simulink model "PC_MSFS_STATION"  (R2021b)
settings: Solver=FixedStepAuto  StartTime=0.0  StopTime=600  FixedStep=0.03  RelTol=1e-3
undefined symbols (not defined in the file): DiscIntNeverNeededParam, MODEL, MODEL_INI
libraries: SimConnectToolbox x9, simulink x4
(part 1 of 2)
settings Model: Creator=Andreas  LastModifiedBy=ccortes9
settings SolverCC: AlgebraicLoopSolver=TrustRegion
settings DebuggingCC: InheritedTsInSrcMsg=none  SFMachineParentedDataDiag=warning

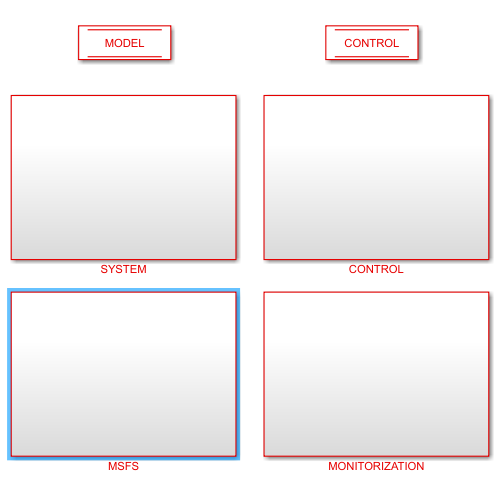
[thumbnail: Simulink's stored preview of the top-level diagram]
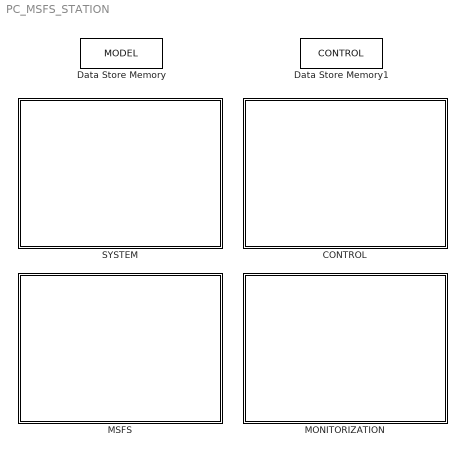
== system PC_MSFS_STATION ==
  CONTROL : Subsystem
  Data Store Memory : DataStoreMemory  DataStoreName=MODEL  ReadBeforeWriteMsg=warning  WriteAfterWriteMsg=warning  WriteAfterReadMsg=warning  InitialValue=MODEL_INI  ShowAdditionalParam=off  OutDataTypeStr=Bus: MODEL_Bus
  Data Store Memory1 : DataStoreMemory  DataStoreName=CONTROL  ReadBeforeWriteMsg=warning  WriteAfterWriteMsg=warning  WriteAfterReadMsg=warning  InitialValue=CONTROL_INI  ShowAdditionalParam=off  OutDataTypeStr=Bus: CONTROL_Bus
  MONITORIZATION : Subsystem
  MSFS : Subsystem
  SYSTEM : Subsystem

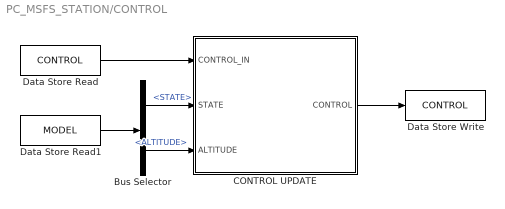
== system PC_MSFS_STATION/CONTROL ==
  Bus Selector : BusSelector  OutputSignals=STATE,INPUT.ALTITUDE
  CONTROL UPDATE : MATLAB Function  TreatAsAtomicUnit=on
  Data Store Read : DataStoreRead  DataStoreName=CONTROL  SampleTime=MODEL_INI.PARAM.SIM_SAMPLING_TIME  IndexOptions=Index vector (dialog)  Indices=1  OutputSizes=1
  Data Store Read1 : DataStoreRead  DataStoreName=MODEL  SampleTime=MODEL_INI.PARAM.SIM_SAMPLING_TIME  IndexOptions=Index vector (dialog)  Indices=1  OutputSizes=1
  Data Store Write : DataStoreWrite  DataStoreName=CONTROL  IndexOptions=Index vector (dialog)  Indices=1  OutputSizes=1
  wires:
  Data Store Read/1 -> CONTROL UPDATE/1(CONTROL_IN)
  CONTROL UPDATE/1(CONTROL) -> Data Store Write/1
  Bus Selector/1 -> CONTROL UPDATE/2(STATE)  "<STATE>"
  Data Store Read1/1 -> Bus Selector/1
  Bus Selector/2 -> CONTROL UPDATE/3(ALTITUDE)  "<ALTITUDE>"

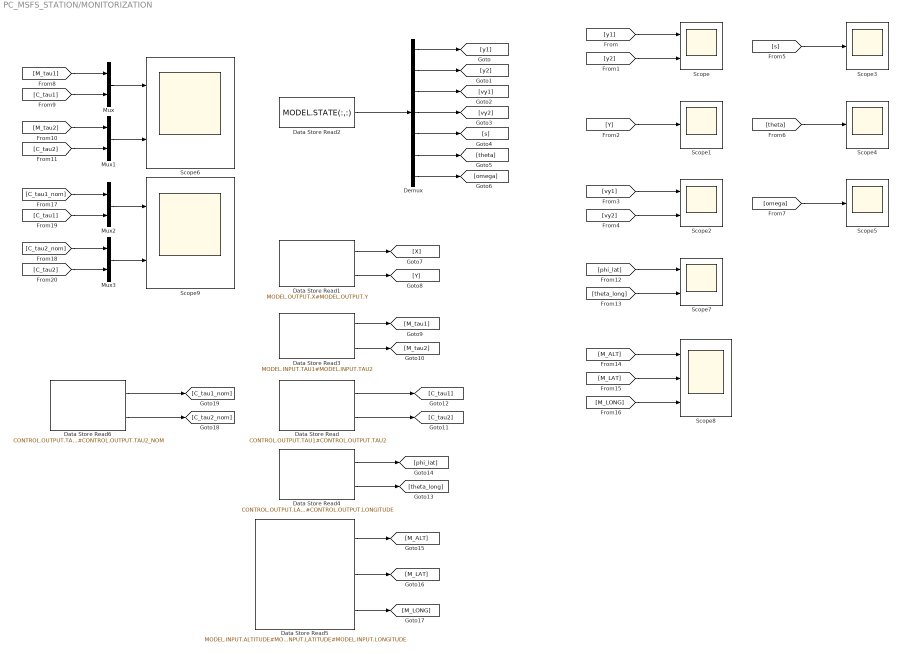
== system PC_MSFS_STATION/MONITORIZATION ==
  Data Store Read : DataStoreRead  DataStoreName=CONTROL  DataStoreElements=CONTROL.OUTPUT.TAU1#CONTROL.OUTPUT.TAU2  IndexOptions=Index vector (dialog)  Indices=1  OutputSizes=1
  Data Store Read1 : DataStoreRead  DataStoreName=MODEL  SampleTime=MODEL_INI.PARAM.SIM_SAMPLING_TIME  DataStoreElements=MODEL.OUTPUT.X#MODEL.OUTPUT.Y  IndexOptions=Index vector (dialog)  Indices=1  OutputSizes=1
  Data Store Read2 : DataStoreRead  DataStoreName=MODEL  SampleTime=MODEL_INI.PARAM.SIM_SAMPLING_TIME  DataStoreElements=MODEL.STATE(:,:)  IndexOptions=Index vector (dialog)  Indices=1  OutputSizes=1
  Data Store Read3 : DataStoreRead  DataStoreName=MODEL  SampleTime=MODEL_INI.PARAM.SIM_SAMPLING_TIME  DataStoreElements=MODEL.INPUT.TAU1#MODEL.INPUT.TAU2  IndexOptions=Index vector (dialog)  Indices=1  OutputSizes=1
  Data Store Read4 : DataStoreRead  DataStoreName=CONTROL  DataStoreElements=CONTROL.OUTPUT.LATITUDE#CONTROL.OUTPUT.LONGITUDE  IndexOptions=Index vector (dialog)  Indices=1  OutputSizes=1
  Data Store Read5 : DataStoreRead  DataStoreName=MODEL  SampleTime=MODEL_INI.PARAM.SIM_SAMPLING_TIME  DataStoreElements=MODEL.INPUT.ALTITUDE#MODEL.INPUT.LATITUDE#MODEL.INPUT.LONGITUDE  IndexOptions=Index vector (dialog)  Indices=1  OutputSizes=1
  Data Store Read6 : DataStoreRead  DataStoreName=CONTROL  DataStoreElements=CONTROL.OUTPUT.TAU1_NOM#CONTROL.OUTPUT.TAU2_NOM  IndexOptions=Index vector (dialog)  Indices=1  OutputSizes=1
  Demux : Demux  Outputs=7
  Mux{,1..3} (4 alike) : Mux  Inputs=2
  Scope{,2,6..7,9} (5 alike) : Scope  NumInputPorts=2
  Scope{1,3..5} (4 alike) : Scope
  Scope8 : Scope  NumInputPorts=3
  wires:
  Data Store Read2/1 -> Demux/1
  Demux/1 -> [y1]
  Demux/2 -> [y2]
  Demux/3 -> [vy1]
  Demux/4 -> [vy2]
  Demux/5 -> [s]
  Demux/6 -> [theta]
  Demux/7 -> [omega]
  [y1] -> Scope/1
  [y2] -> Scope/2
  Data Store Read1/1 -> [X]
  Data Store Read1/2 -> [Y]
  [Y] -> Scope1/1
  [vy2] -> Scope2/2
  [vy1] -> Scope2/1
  [s] -> Scope3/1
  [theta] -> Scope4/1
  [omega] -> Scope5/1
  Data Store Read3/1 -> [M_tau1]
  Data Store Read3/2 -> [M_tau2]
  Data Store Read/1 -> [C_tau1]
  Data Store Read/2 -> [C_tau2]
  Mux/1 -> Scope6/1
  Mux1/1 -> Scope6/2
  [M_tau1] -> Mux/1
  [M_tau2] -> Mux1/1
  [C_tau2] -> Mux1/2
  [C_tau1] -> Mux/2
  [phi_lat] -> Scope7/1
  [theta_long] -> Scope7/2
  Data Store Read4/2 -> [theta_long]
  Data Store Read4/1 -> [phi_lat]
  Data Store Read5/2 -> [M_LAT]
  Data Store Read5/1 -> [M_ALT]
  Data Store Read5/3 -> [M_LONG]
  [M_LAT] -> Scope8/2
  [M_ALT] -> Scope8/1
  [M_LONG] -> Scope8/3
  Data Store Read6/2 -> [C_tau2_nom]
  Data Store Read6/1 -> [C_tau1_nom]
  [C_tau1] -> Mux2/2
  [C_tau2] -> Mux3/2
  [C_tau2_nom] -> Mux3/1
  [C_tau1_nom] -> Mux2/1
  Mux3/1 -> Scope9/2
  Mux2/1 -> Scope9/1

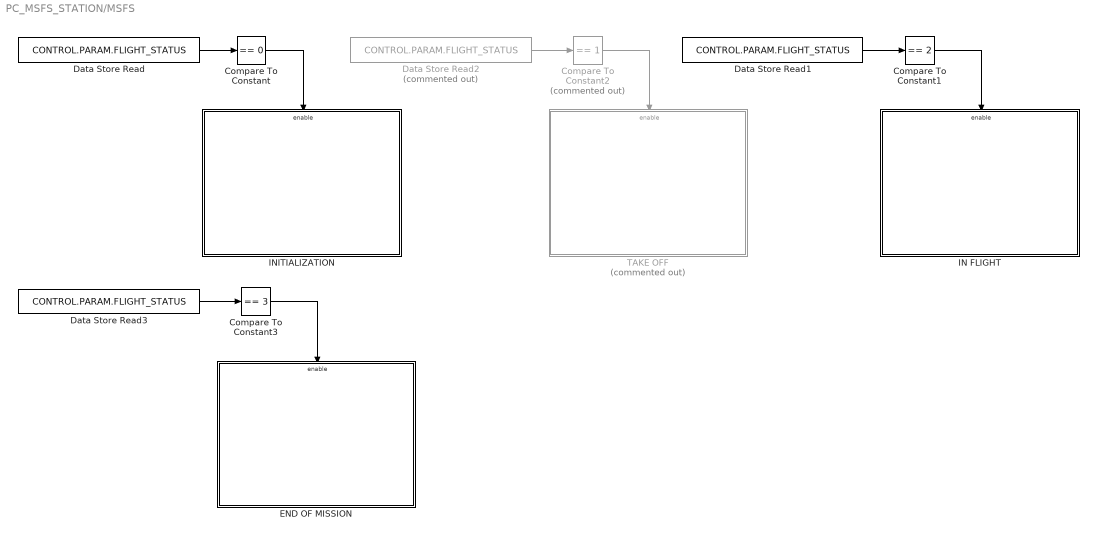
== system PC_MSFS_STATION/MSFS ==
  Compare To Constant : simulink/Logic and Bit Operations/Compare To Constant  relop===  const=0  OutDataTypeStr=boolean
  Compare To Constant1 : simulink/Logic and Bit Operations/Compare To Constant  relop===  const=2  OutDataTypeStr=boolean
  Compare To Constant2 : simulink/Logic and Bit Operations/Compare To Constant  Commented=on  relop===  const=1  OutDataTypeStr=boolean
  Compare To Constant3 : simulink/Logic and Bit Operations/Compare To Constant  relop===  const=3  OutDataTypeStr=boolean
  Data Store Read : DataStoreRead  DataStoreName=CONTROL  DataStoreElements=CONTROL.PARAM.FLIGHT_STATUS  IndexOptions=Index vector (dialog)  Indices=1  OutputSizes=1
  Data Store Read1 : DataStoreRead  DataStoreName=CONTROL  DataStoreElements=CONTROL.PARAM.FLIGHT_STATUS  IndexOptions=Index vector (dialog)  Indices=1  OutputSizes=1
  Data Store Read2 : DataStoreRead  Commented=on  DataStoreName=CONTROL  DataStoreElements=CONTROL.PARAM.FLIGHT_STATUS  IndexOptions=Index vector (dialog)  Indices=1  OutputSizes=1
  Data Store Read3 : DataStoreRead  DataStoreName=CONTROL  DataStoreElements=CONTROL.PARAM.FLIGHT_STATUS  IndexOptions=Index vector (dialog)  Indices=1  OutputSizes=1
  END OF MISSION : Subsystem
  IN FLIGHT : Subsystem
  INITIALIZATION : Subsystem
  TAKE OFF : Subsystem  Commented=on
  wires:
  Data Store Read/1 -> Compare To Constant/1
  Compare To Constant/1 -> INITIALIZATION/Enable
  Data Store Read1/1 -> Compare To Constant1/1
  Compare To Constant1/1 -> IN FLIGHT/Enable
  Data Store Read2/1 -> Compare To Constant2/1
  Compare To Constant2/1 -> TAKE OFF/Enable
  Compare To Constant3/1 -> END OF MISSION/Enable
  Data Store Read3/1 -> Compare To Constant3/1

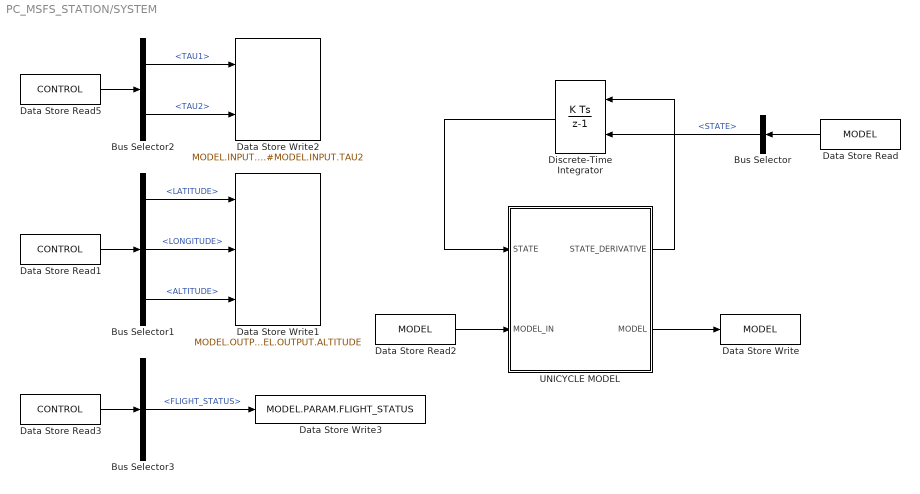
== system PC_MSFS_STATION/SYSTEM ==
  Bus Selector : BusSelector  OutputSignals=STATE
  Bus Selector1 : BusSelector  OutputSignals=OUTPUT.LATITUDE,OUTPUT.LONGITUDE,PARAM.ALTITUDE
  Bus Selector2 : BusSelector  OutputSignals=OUTPUT.TAU1,OUTPUT.TAU2
  Bus Selector3 : BusSelector  OutputSignals=PARAM.FLIGHT_STATUS
  Data Store Read : DataStoreRead  DataStoreName=MODEL  SampleTime=MODEL_INI.PARAM.SIM_SAMPLING_TIME  IndexOptions=Index vector (dialog)  Indices=1  OutputSizes=1
  Data Store Read1 : DataStoreRead  DataStoreName=CONTROL  IndexOptions=Index vector (dialog)  Indices=1  OutputSizes=1
  Data Store Read2 : DataStoreRead  DataStoreName=MODEL  SampleTime=MODEL_INI.PARAM.SIM_SAMPLING_TIME  IndexOptions=Index vector (dialog)  Indices=1  OutputSizes=1
  Data Store Read3 : DataStoreRead  DataStoreName=CONTROL  IndexOptions=Index vector (dialog)  Indices=1  OutputSizes=1
  Data Store Read5 : DataStoreRead  DataStoreName=CONTROL  IndexOptions=Index vector (dialog)  Indices=1  OutputSizes=1
  Data Store Write : DataStoreWrite  DataStoreName=MODEL  IndexOptions=Index vector (dialog)  Indices=1  OutputSizes=1
  Data Store Write1 : DataStoreWrite  DataStoreName=MODEL  DataStoreElements=MODEL.OUTPUT.LATITUDE#MODEL.OUTPUT.LONGITUDE#MODEL.OUTPUT.ALTITUDE  IndexOptions=Index vector (dialog)  Indices=1  OutputSizes=1
  Data Store Write2 : DataStoreWrite  DataStoreName=MODEL  DataStoreElements=MODEL.INPUT.TAU1#MODEL.INPUT.TAU2  IndexOptions=Index vector (dialog)  Indices=1  OutputSizes=1
  Data Store Write3 : DataStoreWrite  DataStoreName=MODEL  DataStoreElements=MODEL.PARAM.FLIGHT_STATUS  IndexOptions=Index vector (dialog)  Indices=1  OutputSizes=1
  Discrete-Time Integrator : DiscreteIntegrator  InitialConditionSource=external  SampleTime=-1  ICPrevOutput=DiscIntNeverNeededParam  ICPrevScaledInput=DiscIntNeverNeededParam
  UNICYCLE MODEL : MATLAB Function  TreatAsAtomicUnit=on
  wires:
  Discrete-Time Integrator/1 -> UNICYCLE MODEL/1(STATE)
  UNICYCLE MODEL/1(STATE_DERIVATIVE) -> Discrete-Time Integrator/1
  Bus Selector/1 -> Discrete-Time Integrator/2  "<STATE>"
  Data Store Read/1 -> Bus Selector/1
  Data Store Read2/1 -> UNICYCLE MODEL/2(MODEL_IN)
  UNICYCLE MODEL/2(MODEL) -> Data Store Write/1
  Bus Selector2/2 -> Data Store Write2/2  "<TAU2>"
  Bus Selector2/1 -> Data Store Write2/1  "<TAU1>"
  Data Store Read5/1 -> Bus Selector2/1
  Data Store Read1/1 -> Bus Selector1/1
  Bus Selector1/1 -> Data Store Write1/1  "<LATITUDE>"
  Bus Selector1/2 -> Data Store Write1/2  "<LONGITUDE>"
  Bus Selector1/3 -> Data Store Write1/3  "<ALTITUDE>"
  Data Store Read3/1 -> Bus Selector3/1
  Bus Selector3/1 -> Data Store Write3/1  "<FLIGHT_STATUS>"

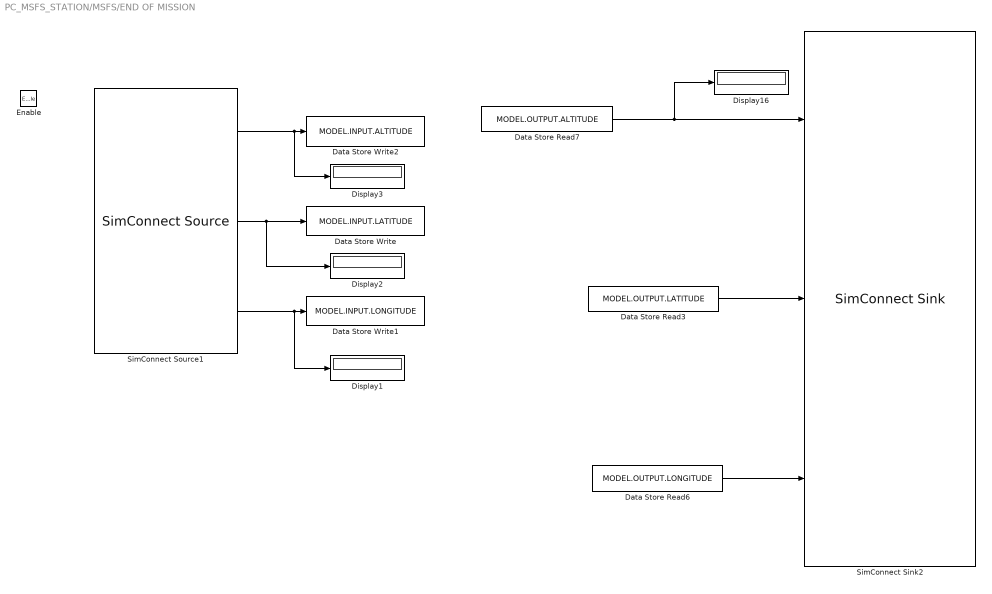
== system PC_MSFS_STATION/MSFS/END OF MISSION ==
  Enable : EnablePort
  Data Store Read3 : DataStoreRead  DataStoreName=MODEL  DataStoreElements=MODEL.OUTPUT.LATITUDE  IndexOptions=Index vector (dialog)  Indices=1  OutputSizes=1
  Data Store Read6 : DataStoreRead  DataStoreName=MODEL  DataStoreElements=MODEL.OUTPUT.LONGITUDE  IndexOptions=Index vector (dialog)  Indices=1  OutputSizes=1
  Data Store Read7 : DataStoreRead  DataStoreName=MODEL  DataStoreElements=MODEL.OUTPUT.ALTITUDE  IndexOptions=Index vector (dialog)  Indices=1  OutputSizes=1
  Data Store Write : DataStoreWrite  DataStoreName=MODEL  DataStoreElements=MODEL.INPUT.LATITUDE  IndexOptions=Index vector (dialog)  Indices=1  OutputSizes=1
  Data Store Write1 : DataStoreWrite  DataStoreName=MODEL  DataStoreElements=MODEL.INPUT.LONGITUDE  IndexOptions=Index vector (dialog)  Indices=1  OutputSizes=1
  Data Store Write2 : DataStoreWrite  DataStoreName=MODEL  DataStoreElements=MODEL.INPUT.ALTITUDE  IndexOptions=Index vector (dialog)  Indices=1  OutputSizes=1
  Display{1..3,16} (4 alike) : Display
  SimConnect Sink2 : SimConnectToolbox/SimConnect Sink  configurationIndex=0  connectionName=SimConnectSink  variables=|
      | PLANE ALTITUDE, FEET;
      | PLANE LATITUDE, RADIANS;
      | PLANE LONGITUDE, RADIANS;
      settings: SourceProductName=SimConnect Toolbox
      mask Display:
      | % This is a new mask on top of the base mask.
      | % Use "View base mask" link below to see the base mask.
      | %port_label('input', 1, 'Rudder Trim', 'texmode', 'on')
      | port_label('input', 1, 'PLANE ALTITUDE, FEET', 'texmode', 'on')
      | port_label('input', 2, 'PLANE LATITUDE, RADIANS', 'texmode', 'on')
      | port_label('input', 3, 'PLANE LONGITUDE, RADIANS', 'texmode', 'on')
  SimConnect Source1 : SimConnectToolbox/SimConnect Source  configurationIndex=0  connectionName=SimConnectSource  variables=|
      | PLANE ALTITUDE, FEET;
      | PLANE LATITUDE, RADIANS;
      | PLANE LONGITUDE, RADIANS;
      settings: SourceProductName=SimConnect Toolbox
      mask Display:
      | % This is a new mask on top of the base mask.
      | % Use "View base mask" link below to see the base mask.
      | % port_label('output', 1, 'g', 'texmode', 'on')
      | port_label('output', 1, 'PLANE ALTITUDE, FEET', 'texmode', 'on')
      | port_label('output', 2, 'PLANE LATITUDE, RADIANS', 'texmode', 'on')
      | port_label('output', 3, 'PLANE LONGITUDE, RADIANS', 'texmode', 'on')
  wires:
  SimConnect Source1/3 -> Display1/1, Data Store Write1/1
  SimConnect Source1/1 -> Display3/1, Data Store Write2/1
  SimConnect Source1/2 -> Display2/1, Data Store Write/1
  Data Store Read7/1 -> Display16/1, SimConnect Sink2/1
  Data Store Read6/1 -> SimConnect Sink2/3
  Data Store Read3/1 -> SimConnect Sink2/2

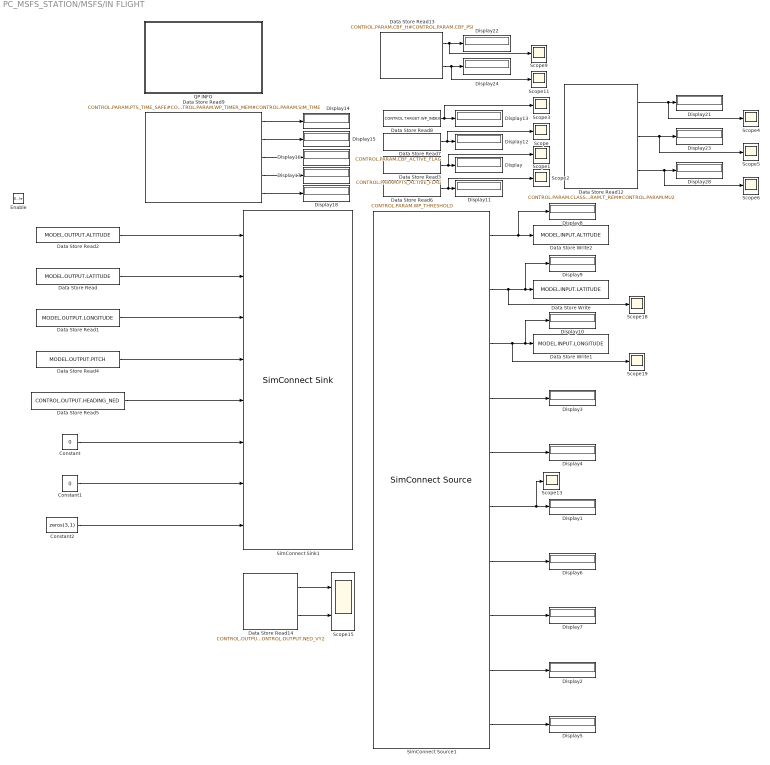
== system PC_MSFS_STATION/MSFS/IN FLIGHT ==
  Enable : EnablePort
  Constant : Constant  Value=0  SampleTime=-1
  Constant1 : Constant  Value=0  SampleTime=-1
  Constant2 : Constant  Value=zeros(3,1)  SampleTime=-1
  Data Store Read : DataStoreRead  DataStoreName=MODEL  DataStoreElements=MODEL.OUTPUT.LATITUDE  IndexOptions=Index vector (dialog)  Indices=1  OutputSizes=1
  Data Store Read1 : DataStoreRead  DataStoreName=MODEL  DataStoreElements=MODEL.OUTPUT.LONGITUDE  IndexOptions=Index vector (dialog)  Indices=1  OutputSizes=1
  Data Store Read12 : DataStoreRead  DataStoreName=CONTROL  DataStoreElements=CONTROL.PARAM.CLASSK#CONTROL.PARAM.T_REM#CONTROL.PARAM.MU2  IndexOptions=Index vector (dialog)  Indices=1  OutputSizes=1
  Data Store Read13 : DataStoreRead  DataStoreName=CONTROL  DataStoreElements=CONTROL.PARAM.CBF_H#CONTROL.PARAM.CBF_PSI  IndexOptions=Index vector (dialog)  Indices=1  OutputSizes=1
  Data Store Read14 : DataStoreRead  DataStoreName=CONTROL  DataStoreElements=CONTROL.OUTPUT.NED_VY1#CONTROL.OUTPUT.NED_VY2  IndexOptions=Index vector (dialog)  Indices=1  OutputSizes=1
  Data Store Read2 : DataStoreRead  DataStoreName=MODEL  DataStoreElements=MODEL.OUTPUT.ALTITUDE  IndexOptions=Index vector (dialog)  Indices=1  OutputSizes=1
  Data Store Read3 : DataStoreRead  DataStoreName=CONTROL  DataStoreElements=CONTROL.PARAM.PTS_ACTIVE_FLAG  IndexOptions=Index vector (dialog)  Indices=1  OutputSizes=1
  Data Store Read4 : DataStoreRead  DataStoreName=MODEL  DataStoreElements=MODEL.OUTPUT.PITCH  IndexOptions=Index vector (dialog)  Indices=1  OutputSizes=1
  Data Store Read5 : DataStoreRead  DataStoreName=CONTROL  DataStoreElements=CONTROL.OUTPUT.HEADING_NED  IndexOptions=Index vector (dialog)  Indices=1  OutputSizes=1
  Data Store Read6 : DataStoreRead  DataStoreName=CONTROL  DataStoreElements=CONTROL.PARAM.WP_THRESHOLD  IndexOptions=Index vector (dialog)  Indices=1  OutputSizes=1
  Data Store Read7 : DataStoreRead  DataStoreName=CONTROL  DataStoreElements=CONTROL.PARAM.CBF_ACTIVE_FLAG  IndexOptions=Index vector (dialog)  Indices=1  OutputSizes=1
  Data Store Read8 : DataStoreRead  DataStoreName=CONTROL  DataStoreElements=CONTROL.TARGET.WP_INDEX  IndexOptions=Index vector (dialog)  Indices=1  OutputSizes=1
  Data Store Read9 : DataStoreRead  DataStoreName=CONTROL  DataStoreElements=CONTROL.PARAM.PTS_TIME_SAFE#CONTROL.PARAM.TIMER#CONTROL.PARAM.WP_TIMER#CONTROL.PARAM.WP_TIMER_MEM#CONTROL.PARAM.SIM_TIME  IndexOptions=Index vector (dialog)  Indices=1  OutputSizes=1
  Data Store Write : DataStoreWrite  DataStoreName=MODEL  DataStoreElements=MODEL.INPUT.LATITUDE  IndexOptions=Index vector (dialog)  Indices=1  OutputSizes=1
  Data Store Write1 : DataStoreWrite  DataStoreName=MODEL  DataStoreElements=MODEL.INPUT.LONGITUDE  IndexOptions=Index vector (dialog)  Indices=1  OutputSizes=1
  Data Store Write2 : DataStoreWrite  DataStoreName=MODEL  DataStoreElements=MODEL.INPUT.ALTITUDE  IndexOptions=Index vector (dialog)  Indices=1  OutputSizes=1
  Display{,1..18,21..24,28} (24 alike) : Display
  QP INFO : Subsystem
  Scope{,1..6,9,11,13,18..19} (12 alike) : Scope
  Scope15 : Scope  NumInputPorts=2
  SimConnect Sink1 : SimConnectToolbox/SimConnect Sink  configurationIndex=0  connectionName=SimConnectSink  variables=|
      | PLANE ALTITUDE, FEET;
      | PLANE LATITUDE, RADIANS;
      | PLANE LONGITUDE, RADIANS;
      | PLANE PITCH DEGREES, RADIANS;
      | PLANE HEADING DEGREES TRUE, RADIANS;
      | ROTATION VELOCITY BODY X, FEET PER SECOND;
      | AILERON POSITION, POSITION;
      | AILERON TRIM PCT, PERCENT;
      settings: SourceProductName=SimConnect Toolbox
      mask Display:
      | % This is a new mask on top of the base mask.
      | % Use "View base mask" link below to see the base mask.
      | %port_label('input', 1, 'Rudder Trim', 'texmode', 'on')
      | port_label('input', 1, 'PLANE ALTITUDE, FEET', 'texmode', 'on')
      | port_label('input', 2, 'PLANE LATITUDE, RADIANS', 'texmode', 'on')
      | port_label('input', 3, 'PLANE LONGITUDE, RADIANS', 'texmode', 'on')
      | port_label('input', 4, 'PITCH DEGREES, RADIANS', 'texmode', 'on')
      | port_label('input', 5, 'HEADING DEGREES TRUE, RADIANS', 'texmode', 'on')
      | port_label('input', 6, 'VELOCITY BODY X, FEET PER SECOND', 'texmode', 'on')
      | port_label('input', 7, 'AILERON POSITION, POSITION', 'texmode', 'on')
      | port_label('input', 8, 'AILERON TRIM PCT, PERCENT OVER 100', 'texmode', 'on')
  SimConnect Source1 : SimConnectToolbox/SimConnect Source  configurationIndex=0  connectionName=SimConnectSource  variables=|
      | PLANE ALTITUDE, FEET;
      | PLANE LATITUDE, RADIANS;
      | PLANE LONGITUDE, RADIANS;
      | ROTATION VELOCITY BODY X, FEET PER SECOND;
      | PLANE PITCH DEGREES, RADIANS;
      | PLANE HEADING DEGREES TRUE, RADIANS;
      | PLANE HEADING DEGREES MAGNETIC, RADIANS;
      | PLANE HEADING DEGREES GYRO, DEGREES;
      | AILERON POSITION, POSITION;
      | AILERON TRIM PCT, PERCENT OVER 100;
      settings: SourceProductName=SimConnect Toolbox
      mask Display:
      | % This is a new mask on top of the base mask.
      | % Use "View base mask" link below to see the base mask.
      | % port_label('output', 1, 'g', 'texmode', 'on')
      | port_label('output', 1, 'PLANE ALTITUDE, FEET', 'texmode', 'on')
      | port_label('output', 2, 'PLANE LATITUDE, RADIANS', 'texmode', 'on')
      | port_label('output', 3, 'PLANE LONGITUDE, RADIANS', 'texmode', 'on')
      | port_label('output', 4, 'VELOCITY BODY X, FEET PER SECOND', 'texmode', 'on')
      | port_label('output', 5, 'PITCH DEGREES, RADIANS', 'texmode', 'on')
      | port_label('output', 6, 'HEADING DEGREES TRUE, RADIANS', 'texmode', 'on')
      | port_label('output', 7, 'HEADING DEGREES MAGNETIC, RADIANS', 'texmode', 'on')
      | port_label('output', 8, 'HEADING DEGREES GYRO, DEGREES', 'texmode', 'on')
      | port_label('output', 9, 'AILERON POSITION, POSITION', 'texmode', 'on')
      | port_label('output', 10, 'AILERON TRIM PCT, PERCENT OVER 100', 'texmode', 'on')
  wires:
  Constant2/1 -> SimConnect Sink1/8
  SimConnect Source1/9 -> Display2/1
  Constant/1 -> SimConnect Sink1/6
  Data Store Read1/1 -> SimConnect Sink1/3
  Constant1/1 -> SimConnect Sink1/7
  SimConnect Source1/5 -> Display4/1
  SimConnect Source1/3 -> Scope19/1, Display10/1, Data Store Write1/1
  SimConnect Source1/2 -> Scope18/1, Display9/1, Data Store Write/1
  SimConnect Source1/8 -> Display7/1
  SimConnect Source1/6 -> Scope13/1, Display1/1
  Data Store Read2/1 -> SimConnect Sink1/1
  Data Store Read/1 -> SimConnect Sink1/2
  Data Store Read4/1 -> SimConnect Sink1/4
  SimConnect Source1/4 -> Display3/1
  SimConnect Source1/1 -> Display8/1, Data Store Write2/1
  SimConnect Source1/7 -> Display6/1
  SimConnect Source1/10 -> Display5/1
  Data Store Read3/1 -> Scope1/1, Display/1
  Data Store Read6/1 -> Scope2/1, Display11/1
  Data Store Read7/1 -> Scope/1, Display12/1
  Data Store Read8/1 -> Scope3/1, Display13/1
  Data Store Read9/1 -> Display14/1
  Data Store Read9/2 -> Display15/1
  Data Store Read9/3 -> Display16/1
  Data Store Read9/4 -> Display17/1
  Data Store Read9/5 -> Display18/1
  Data Store Read13/1 -> Display22/1, Scope9/1
  Data Store Read13/2 -> Display24/1, Scope11/1
  Data Store Read14/1 -> Scope15/1
  Data Store Read14/2 -> Scope15/2
  Data Store Read5/1 -> SimConnect Sink1/5
  Data Store Read12/1 -> Scope4/1, Display21/1
  Data Store Read12/2 -> Scope5/1, Display23/1
  Data Store Read12/3 -> Scope6/1, Display28/1

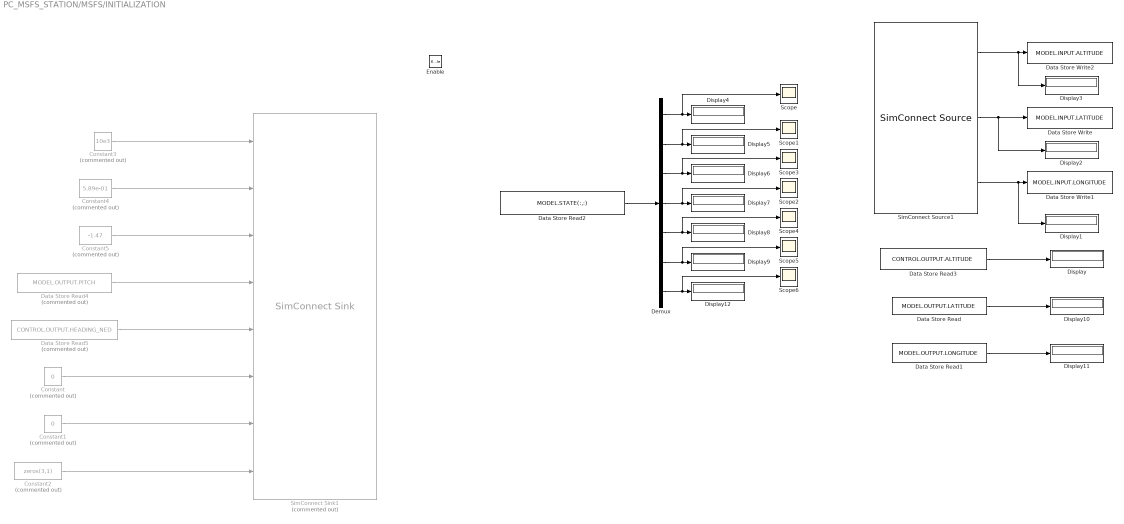
== system PC_MSFS_STATION/MSFS/INITIALIZATION ==
  Enable : EnablePort
  Constant : Constant  Commented=on  Value=0  SampleTime=-1
  Constant1 : Constant  Commented=on  Value=0  SampleTime=-1
  Constant2 : Constant  Commented=on  Value=zeros(3,1)  SampleTime=-1
  Constant3 : Constant  Commented=on  Value=10e3  SampleTime=-1
  Constant4 : Constant  Commented=on  Value=5.89e-01  SampleTime=-1
  Constant5 : Constant  Commented=on  Value=-1.47  SampleTime=-1
  Data Store Read : DataStoreRead  DataStoreName=MODEL  DataStoreElements=MODEL.OUTPUT.LATITUDE  IndexOptions=Index vector (dialog)  Indices=1  OutputSizes=1
  Data Store Read1 : DataStoreRead  DataStoreName=MODEL  DataStoreElements=MODEL.OUTPUT.LONGITUDE  IndexOptions=Index vector (dialog)  Indices=1  OutputSizes=1
  Data Store Read2 : DataStoreRead  DataStoreName=MODEL  DataStoreElements=MODEL.STATE(:,:)  IndexOptions=Index vector (dialog)  Indices=1  OutputSizes=1
  Data Store Read3 : DataStoreRead  DataStoreName=CONTROL  DataStoreElements=CONTROL.OUTPUT.ALTITUDE  IndexOptions=Index vector (dialog)  Indices=1  OutputSizes=1
  Data Store Read4 : DataStoreRead  Commented=on  DataStoreName=MODEL  DataStoreElements=MODEL.OUTPUT.PITCH  IndexOptions=Index vector (dialog)  Indices=1  OutputSizes=1
  Data Store Read5 : DataStoreRead  Commented=on  DataStoreName=CONTROL  DataStoreElements=CONTROL.OUTPUT.HEADING_NED  IndexOptions=Index vector (dialog)  Indices=1  OutputSizes=1
  Data Store Write : DataStoreWrite  DataStoreName=MODEL  DataStoreElements=MODEL.INPUT.LATITUDE  IndexOptions=Index vector (dialog)  Indices=1  OutputSizes=1
  Data Store Write1 : DataStoreWrite  DataStoreName=MODEL  DataStoreElements=MODEL.INPUT.LONGITUDE  IndexOptions=Index vector (dialog)  Indices=1  OutputSizes=1
  Data Store Write2 : DataStoreWrite  DataStoreName=MODEL  DataStoreElements=MODEL.INPUT.ALTITUDE  IndexOptions=Index vector (dialog)  Indices=1  OutputSizes=1
  Demux : Demux  Outputs=7
  Display{,1..12} (13 alike) : Display
  Scope{,1..6} (7 alike) : Scope
  SimConnect Sink1 : SimConnectToolbox/SimConnect Sink  Commented=on  configurationIndex=0  connectionName=SimConnectSink  variables=|
      | PLANE ALTITUDE, FEET;
      | PLANE LATITUDE, RADIANS;
      | PLANE LONGITUDE, RADIANS;
      | PLANE PITCH DEGREES, RADIANS;
      | PLANE HEADING DEGREES TRUE, RADIANS;
      | ROTATION VELOCITY BODY X, FEET PER SECOND;
      | AILERON POSITION, POSITION;
      | AILERON TRIM PCT, PERCENT;
      settings: SourceProductName=SimConnect Toolbox
      mask Display:
      | % This is a new mask on top of the base mask.
      | % Use "View base mask" link below to see the base mask.
      | %port_label('input', 1, 'Rudder Trim', 'texmode', 'on')
      | port_label('input', 1, 'PLANE ALTITUDE, FEET', 'texmode', 'on')
      | port_label('input', 2, 'PLANE LATITUDE, RADIANS', 'texmode', 'on')
      | port_label('input', 3, 'PLANE LONGITUDE, RADIANS', 'texmode', 'on')
      | port_label('input', 4, 'PITCH DEGREES, RADIANS', 'texmode', 'on')
      | port_label('input', 5, 'HEADING DEGREES TRUE, RADIANS', 'texmode', 'on')
      | port_label('input', 6, 'VELOCITY BODY X, FEET PER SECOND', 'texmode', 'on')
      | port_label('input', 7, 'AILERON POSITION, POSITION', 'texmode', 'on')
      | port_label('input', 8, 'AILERON TRIM PCT, PERCENT OVER 100', 'texmode', 'on')
  SimConnect Source1 : SimConnectToolbox/SimConnect Source  configurationIndex=0  connectionName=SimConnectSource  variables=|
      | PLANE ALTITUDE, FEET;
      | PLANE LATITUDE, RADIANS;
      | PLANE LONGITUDE, RADIANS;
      settings: SourceProductName=SimConnect Toolbox
      mask Display:
      | % This is a new mask on top of the base mask.
      | % Use "View base mask" link below to see the base mask.
      | % port_label('output', 1, 'g', 'texmode', 'on')
      | port_label('output', 1, 'PLANE ALTITUDE, FEET', 'texmode', 'on')
      | port_label('output', 2, 'PLANE LATITUDE, RADIANS', 'texmode', 'on')
      | port_label('output', 3, 'PLANE LONGITUDE, RADIANS', 'texmode', 'on')
  wires:
  Data Store Read4/1 -> SimConnect Sink1/4
  Constant4/1 -> SimConnect Sink1/2
  Constant3/1 -> SimConnect Sink1/1
  Constant1/1 -> SimConnect Sink1/7
  Constant5/1 -> SimConnect Sink1/3
  Constant/1 -> SimConnect Sink1/6
  Data Store Read5/1 -> SimConnect Sink1/5
  Constant2/1 -> SimConnect Sink1/8
  SimConnect Source1/1 -> Display3/1, Data Store Write2/1
  SimConnect Source1/2 -> Display2/1, Data Store Write/1
  SimConnect Source1/3 -> Display1/1, Data Store Write1/1
  Data Store Read1/1 -> Display11/1
  Data Store Read3/1 -> Display/1
  Data Store Read/1 -> Display10/1
  Data Store Read2/1 -> Demux/1
  Demux/1 -> Scope/1, Display4/1
  Demux/2 -> Scope1/1, Display5/1
  Demux/3 -> Scope3/1, Display6/1
  Demux/4 -> Scope2/1, Display7/1
  Demux/5 -> Scope4/1, Display8/1
  Demux/6 -> Scope5/1, Display9/1
  Demux/7 -> Scope6/1, Display12/1

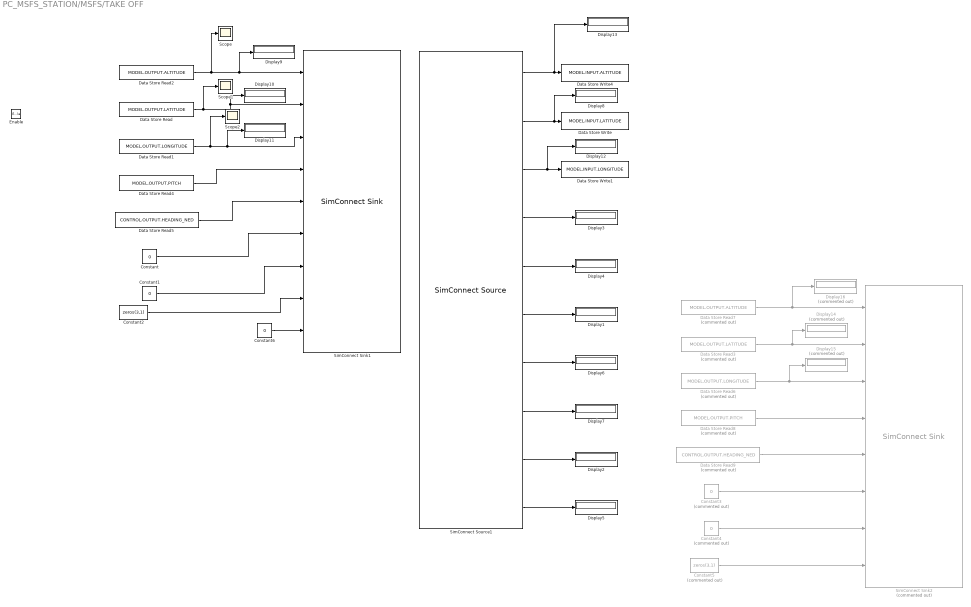
== system PC_MSFS_STATION/MSFS/TAKE OFF ==
  Enable : EnablePort
  Constant : Constant  Value=0  SampleTime=-1
  Constant1 : Constant  Value=0  SampleTime=-1
  Constant2 : Constant  Value=zeros(3,1)  SampleTime=-1
  Constant3 : Constant  Commented=on  Value=0  SampleTime=-1
  Constant4 : Constant  Commented=on  Value=0  SampleTime=-1
  Constant5 : Constant  Commented=on  Value=zeros(3,1)  SampleTime=-1
  Constant6 : Constant  Value=0  SampleTime=-1
  Data Store Read : DataStoreRead  DataStoreName=MODEL  DataStoreElements=MODEL.OUTPUT.LATITUDE  IndexOptions=Index vector (dialog)  Indices=1  OutputSizes=1
  Data Store Read1 : DataStoreRead  DataStoreName=MODEL  DataStoreElements=MODEL.OUTPUT.LONGITUDE  IndexOptions=Index vector (dialog)  Indices=1  OutputSizes=1
  Data Store Read2 : DataStoreRead  DataStoreName=MODEL  DataStoreElements=MODEL.OUTPUT.ALTITUDE  IndexOptions=Index vector (dialog)  Indices=1  OutputSizes=1
  Data Store Read3 : DataStoreRead  Commented=on  DataStoreName=MODEL  DataStoreElements=MODEL.OUTPUT.LATITUDE  IndexOptions=Index vector (dialog)  Indices=1  OutputSizes=1
  Data Store Read4 : DataStoreRead  DataStoreName=MODEL  DataStoreElements=MODEL.OUTPUT.PITCH  IndexOptions=Index vector (dialog)  Indices=1  OutputSizes=1
  Data Store Read5 : DataStoreRead  DataStoreName=CONTROL  DataStoreElements=CONTROL.OUTPUT.HEADING_NED  IndexOptions=Index vector (dialog)  Indices=1  OutputSizes=1
  Data Store Read6 : DataStoreRead  Commented=on  DataStoreName=MODEL  DataStoreElements=MODEL.OUTPUT.LONGITUDE  IndexOptions=Index vector (dialog)  Indices=1  OutputSizes=1
  Data Store Read7 : DataStoreRead  Commented=on  DataStoreName=MODEL  DataStoreElements=MODEL.OUTPUT.ALTITUDE  IndexOptions=Index vector (dialog)  Indices=1  OutputSizes=1
  Data Store Read8 : DataStoreRead  Commented=on  DataStoreName=MODEL  DataStoreElements=MODEL.OUTPUT.PITCH  IndexOptions=Index vector (dialog)  Indices=1  OutputSizes=1
  Data Store Read9 : DataStoreRead  Commented=on  DataStoreName=CONTROL  DataStoreElements=CONTROL.OUTPUT.HEADING_NED  IndexOptions=Index vector (dialog)  Indices=1  OutputSizes=1
  Data Store Write : DataStoreWrite  DataStoreName=MODEL  DataStoreElements=MODEL.INPUT.LATITUDE  IndexOptions=Index vector (dialog)  Indices=1  OutputSizes=1
  Data Store Write1 : DataStoreWrite  DataStoreName=MODEL  DataStoreElements=MODEL.INPUT.LONGITUDE  IndexOptions=Index vector (dialog)  Indices=1  OutputSizes=1
  Data Store Write4 : DataStoreWrite  DataStoreName=MODEL  DataStoreElements=MODEL.INPUT.ALTITUDE  IndexOptions=Index vector (dialog)  Indices=1  OutputSizes=1
  Display{1..13} (13 alike) : Display
  Display14 : Display  Commented=on
  Display15 : Display  Commented=on
  Display16 : Display  Commented=on
  Scope : Scope
  Scope1 : Scope
  Scope2 : Scope
  SimConnect Sink1 : SimConnectToolbox/SimConnect Sink  configurationIndex=0  connectionName=SimConnectSink  variables=|
      | PLANE ALTITUDE, FEET;
      | PLANE LATITUDE, RADIANS;
      | PLANE LONGITUDE, RADIANS;
      | PLANE PITCH DEGREES, RADIANS;
      | PLANE HEADING DEGREES MAGNETIC, RADIANS;
      | ROTATION VELOCITY BODY X, FEET PER SECOND;
      | AILERON POSITION, POSITION;
      | AILERON TRIM PCT, PERCENT;
      | VERTICAL SPEED, FEET PER SECOND;
      settings: SourceProductName=SimConnect Toolbox
      mask Display:
      | % This is a new mask on top of the base mask.
      | % Use "View base mask" link below to see the base mask.
      | %port_label('input', 1, 'Rudder Trim', 'texmode', 'on')
      | port_label('input', 1, 'PLANE ALTITUDE, FEET', 'texmode', 'on')
      | port_label('input', 2, 'PLANE LATITUDE, RADIANS', 'texmode', 'on')
      | port_label('input', 3, 'PLANE LONGITUDE, RADIANS', 'texmode', 'on')
      | port_label('input', 4, 'PITCH DEGREES, RADIANS', 'texmode', 'on')
      | port_label('input', 5, 'HEADING DEGREES TRUE, RADIANS', 'texmode', 'on')
      | port_label('input', 6, 'VELOCITY BODY X, FEET PER SECOND', 'texmode', 'on')
      | port_label('input', 7, 'AILERON POSITION, POSITION', 'texmode', 'on')
      | port_label('input', 8, 'AILERON TRIM PCT, PERCENT OVER 100', 'texmode', 'on')
      | port_label('input', 9, 'VERTICAL SPEED, FEET PER SECOND', 'texmode', 'on')
  SimConnect Sink2 : SimConnectToolbox/SimConnect Sink  Commented=on  configurationIndex=0  connectionName=SimConnectSink  variables=|
      | PLANE ALTITUDE, FEET;
      | PLANE LATITUDE, RADIANS;
      | PLANE LONGITUDE, RADIANS;
      | PLANE PITCH DEGREES, RADIANS;
      | PLANE HEADING DEGREES MAGNETIC, RADIANS;
      | ROTATION VELOCITY BODY X, FEET PER SECOND;
      | AILERON POSITION, POSITION;
      | AILERON TRIM PCT, PERCENT;
      settings: SourceProductName=SimConnect Toolbox
      mask Display:
      | % This is a new mask on top of the base mask.
      | % Use "View base mask" link below to see the base mask.
      | %port_label('input', 1, 'Rudder Trim', 'texmode', 'on')
      | port_label('input', 1, 'PLANE ALTITUDE, FEET', 'texmode', 'on')
      | port_label('input', 2, 'PLANE LATITUDE, RADIANS', 'texmode', 'on')
      | port_label('input', 3, 'PLANE LONGITUDE, RADIANS', 'texmode', 'on')
      | port_label('input', 4, 'PITCH DEGREES, RADIANS', 'texmode', 'on')
      | port_label('input', 5, 'HEADING DEGREES TRUE, RADIANS', 'texmode', 'on')
      | port_label('input', 6, 'VELOCITY BODY X, FEET PER SECOND', 'texmode', 'on')
      | port_label('input', 7, 'AILERON POSITION, POSITION', 'texmode', 'on')
      | port_label('input', 8, 'AILERON TRIM PCT, PERCENT OVER 100', 'texmode', 'on')
  SimConnect Source1 : SimConnectToolbox/SimConnect Source  configurationIndex=0  connectionName=SimConnectSource  variables=|
      | PLANE ALTITUDE, FEET;
      | PLANE LATITUDE, RADIANS;
      | PLANE LONGITUDE, RADIANS;
      | ROTATION VELOCITY BODY X, FEET PER SECOND;
      | PLANE PITCH DEGREES, RADIANS;
      | PLANE HEADING DEGREES TRUE, RADIANS;
      | PLANE HEADING DEGREES MAGNETIC, RADIANS;
      | PLANE HEADING DEGREES GYRO, DEGREES;
      | AILERON POSITION, POSITION;
      | AILERON TRIM PCT, PERCENT OVER 100;
      settings: SourceProductName=SimConnect Toolbox
      mask Display:
      | % This is a new mask on top of the base mask.
      | % Use "View base mask" link below to see the base mask.
      | % port_label('output', 1, 'g', 'texmode', 'on')
      | port_label('output', 1, 'PLANE ALTITUDE, FEET', 'texmode', 'on')
      | port_label('output', 2, 'PLANE LATITUDE, RADIANS', 'texmode', 'on')
      | port_label('output', 3, 'PLANE LONGITUDE, RADIANS', 'texmode', 'on')
      | port_label('output', 4, 'VELOCITY BODY X, FEET PER SECOND', 'texmode', 'on')
      | port_label('output', 5, 'PITCH DEGREES, RADIANS', 'texmode', 'on')
      | port_label('output', 6, 'HEADING DEGREES TRUE, RADIANS', 'texmode', 'on')
      | port_label('output', 7, 'HEADING DEGREES MAGNETIC, RADIANS', 'texmode', 'on')
      | port_label('output', 8, 'HEADING DEGREES GYRO, DEGREES', 'texmode', 'on')
      | port_label('output', 9, 'AILERON POSITION, POSITION', 'texmode', 'on')
      | port_label('output', 10, 'AILERON TRIM PCT, PERCENT OVER 100', 'texmode', 'on')
  wires:
  Constant2/1 -> SimConnect Sink1/8
  SimConnect Source1/9 -> Display2/1
  Data Store Read5/1 -> SimConnect Sink1/5
  Constant/1 -> SimConnect Sink1/6
  Constant1/1 -> SimConnect Sink1/7
  SimConnect Source1/5 -> Display4/1
  SimConnect Source1/3 -> Display12/1, Data Store Write1/1
  SimConnect Source1/2 -> Display8/1, Data Store Write/1
  SimConnect Source1/8 -> Display7/1
  SimConnect Source1/6 -> Display1/1
  Data Store Read4/1 -> SimConnect Sink1/4
  SimConnect Source1/4 -> Display3/1
  SimConnect Source1/7 -> Display6/1
  SimConnect Source1/10 -> Display5/1
  Data Store Read2/1 -> Scope/1, SimConnect Sink1/1, Display9/1
  Data Store Read/1 -> Scope1/1, Display10/1, SimConnect Sink1/2
  Data Store Read1/1 -> Scope2/1, Display11/1, SimConnect Sink1/3
  SimConnect Source1/1 -> Display13/1, Data Store Write4/1
  Constant4/1 -> SimConnect Sink2/7
  Data Store Read9/1 -> SimConnect Sink2/5
  Data Store Read7/1 -> Display16/1, SimConnect Sink2/1
  Constant5/1 -> SimConnect Sink2/8
  Data Store Read8/1 -> SimConnect Sink2/4
  Data Store Read6/1 -> Display15/1, SimConnect Sink2/3
  Constant3/1 -> SimConnect Sink2/6
  Data Store Read3/1 -> Display14/1, SimConnect Sink2/2
  Constant6/1 -> SimConnect Sink1/9

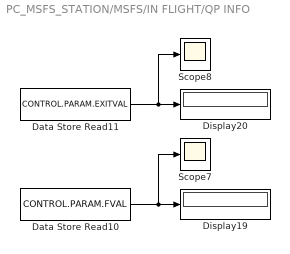
== system PC_MSFS_STATION/MSFS/IN FLIGHT/QP INFO ==
  Data Store Read10 : DataStoreRead  DataStoreName=CONTROL  DataStoreElements=CONTROL.PARAM.FVAL  IndexOptions=Index vector (dialog)  Indices=1  OutputSizes=1
  Data Store Read11 : DataStoreRead  DataStoreName=CONTROL  DataStoreElements=CONTROL.PARAM.EXITVAL  IndexOptions=Index vector (dialog)  Indices=1  OutputSizes=1
  Display19 : Display
  Display20 : Display
  Scope7 : Scope
  Scope8 : Scope
  wires:
  Data Store Read10/1 -> Scope7/1, Display19/1
  Data Store Read11/1 -> Display20/1, Scope8/1

== matlab function PC_MSFS_STATION/CONTROL/CONTROL UPDATE ==
  data: CONTROL_IN input; CONTROL output Bus: CONTROL_Bus; STATE input; ALTITUDE input
function CONTROL = CONTROL_UPDATE(CONTROL_IN, STATE, ALTITUDE)
% COPY CONTROL BUS
CONTROL = CONTROL_IN;
CONTROL.PARAM.SIM_TIME = CONTROL.PARAM.SIM_TIME + CONTROL.PARAM.SAMPLING_TIME;
curr_sim_time = CONTROL.PARAM.SIM_TIME;
deltat = CONTROL.PARAM.SAMPLING_TIME;
flight_status = CONTROL.PARAM.FLIGHT_STATUS;
timer = CONTROL.PARAM.TIMER;

%--------------------------------------------------------------------------
% CONTROL PARAMETERS
%--------------------------------------------------------------------------
% Nominal Control Parameters
kyd = CONTROL.PARAM.NAV_D_1;

% Navigation Variables
altitude = ALTITUDE;
rho = altitude + 20.902e6;
heading = CONTROL.OUTPUT.HEADING;
heading_NED = CONTROL.OUTPUT.HEADING_NED;

% Prescribed Time Safety CBFs
time_PTS_Safe = CONTROL.PARAM.PTS_TIME_SAFE;
PTS_Threshold = CONTROL.PARAM.PTS_THRESHOLD;
PTS_Critical = CONTROL.PARAM.PTS_CRITICAL;
wp_Threshold_Flag = CONTROL.PARAM.WP_THRESHOLD;
time_wp_PTS = CONTROL.PARAM.WP_TIMER;
time_wp_PTS_mem = CONTROL.PARAM.WP_TIMER_MEM;
mu_max = CONTROL.PARAM.MU_MAX;
CBF_const = CONTROL.PARAM.CBF_CONST;
CBF_const2 = CONTROL.PARAM.CBF_CONST2;
t_nu_active = CONTROL.PARAM.TIME_NU_ACT;
PTS_Active = CONTROL.PARAM.PTS_ACTIVE_FLAG;
CBF_active = CONTROL.PARAM.CBF_ACTIVE_FLAG;
h = CONTROL.PARAM.CBF_H;
psi = CONTROL.PARAM.CBF_PSI;

% Extra Parameters
tau_max = CONTROL.PARAM.TAU_MAX;
PTS_Goal = CONTROL.PARAM.PTS_GOAL;


tau1_prev = CONTROL.PARAM.TAU1_PREV;
tau2_prev = CONTROL.PARAM.TAU2_PREV;
fval_qp = CONTROL.PARAM.FVAL;
exitval_qp = CONTROL.PARAM.EXITVAL;
%--------------------------------------------------------------------------
% CONTROL TARGETS
%--------------------------------------------------------------------------
wp_index = CONTROL.TARGET.WP_INDEX;
simu_end = CONTROL.TARGET.SIMU_END;
wp1 = CONTROL.TARGET.TARGET_POS1(wp_index);
wp2 = CONTROL.TARGET.TARGET_POS2(wp_index);
snom = CONTROL.TARGET.VELOCITY;
%--------------------------------------------------------------------------
% SYSTEM CURRENT STATE
%--------------------------------------------------------------------------
% Update Current State
y1 = STATE(1);
y2 = STATE(2);
vy1 = STATE(3);
vy2 = STATE(4);

% % MANUAL TAKEOFF
% if flight_status == 0
%     tau1_applied = 0;
%     tau2_applied = 0;
%     if altitude >= 2*10e2
%         flight_status = 2;
%     end

% AUTOMATIC
if flight_status == 0
    % INITIALIZATION
    tau1_applied = 0;
    tau2_applied = 0;
    tau1_nom_PD = 0;
    tau2_nom_PD = 0;
    if curr_sim_time >= 5
        flight_status = 2;
        altitude = 2*10e2;
        rho = altitude + 20.902e6;
        timer = 0;
    end 

elseif flight_status == 1
    % TAKE OFF
    tau1_applied = - kyd*(vy1 - 0);
    tau2_applied = - kyd*(vy2 - 0);
    tau1_nom_PD = tau1_applied;
    tau2_nom_PD = tau2_applied;
     if abs(tau1_applied) >= tau_max
        tau1_applied = sign(tau1_applied)*tau_max;
    else
        tau1_applied = tau1_applied;
    end

    if abs(tau2_applied) >= tau_max
        tau2_applied = sign(tau2_applied)*tau_max;
    else
        tau2_applied = tau2_applied;
    end
    if timer >= 3
        flight_status = 2;
        timer = 0;
    else
        altitude = 2*10e2;
        rho = altitude + 20.902e6;
        timer = timer + deltat;
    end
elseif flight_status == 2
    % ON FLIGHT
    %--------------------------------------------------------------------------
    % DERIVATIVE (D) CONTROL
    %--------------------------------------------------------------------------
    altitude = 2*10e2;
    rho = altitude + 20.902e6; 
    timer = timer + deltat;
    time_wp_PTS = time_wp_PTS + deltat;

    % UPDATE PTS ACTIVE
    if ((y1 - wp1)^2 + (y2 - wp2)^2 < PTS_Threshold^2)
            if wp_Threshold_Flag == 0
                % System just crossed the threshold
                wp_Threshold_Flag = 1; % Only enters here once
                time_wp_PTS_mem = curr_sim_time; % Save time system crosses threshold
                time_wp_PTS = 0; % Start timer for PTS
            end
            if (time_wp_PTS <= time_PTS_Safe)
                % Safe time hasn't expired
                CBF_active = 1;
                PTS_Active = 1;
            else
                % Safe time has expired
                CBF_active = 0; % System can now reach waypoint
                PTS_Active = 0; 
            end
    end
        
    % BLOW - UP FUNCTION
    if (PTS_Active == 1)
        t_rem = time_PTS_Safe - time_wp_PTS;
        CONTROL.PARAM.T_REM = t_rem;
        if (t_rem <= t_nu_active)
            nu_PTS = time_PTS_Safe/t_nu_active - time_wp_PTS/t_nu_active;
        else
            nu_PTS = 1;
        end
        mu_PTS = 1/nu_PTS;
        if (abs(mu_PTS) >= mu_max)
            mu_PTS = mu_max*sign(mu_PTS);
        end
        mu2_PTS = 1/nu_PTS^2;
        CONTROL.PARAM.MU2 = mu2_PTS;
        if (abs(mu2_PTS) >= mu_max)
            mu2_PTS = mu_max*sign(mu2_PTS);
        end
    else
        nu_PTS = 1;
        mu_PTS = 1;
        mu2_PTS = 1;
    end
    
    % UPDATE TARGET WAYPOINT
    if ((y1 - wp1)^2 + (y2 - wp2)^2 < PTS_Goal^2)
        % UPDATE WAYPOINT INDEX
        wp_index = wp_index + 1;
        % UPDATE SAFETY FILTER PARAMETERS
        CBF_active = 1;
        PTS_Active = 0;
        wp_Threshold_Flag = 0;

        if (wp_index >= 4) % For 3 wp this is a 4
            simu_end = 1;
            CBF_active = 0;
            PTS_Active = 0;
            flight_status = 3;
            wp_index = 3;
%             wp_index = 2;
        end
    end

    % UPDATE TARGET VELOCITY
    if simu_end == 0
        % System Quadrant
        pos1_PD = wp1 - y1;
        pos2_PD = wp2 - y2;

        if pos1_PD >=0
            % First or fourth quadrant
            if pos2_PD >=0
                %First quadrant
                theta_PD = atan(abs(pos2_PD)/abs(pos1_PD));
            else
                % Fourth quadrant
%                 theta_PD = 2*pi - atan(abs(pos2_PD)/abs(pos1_PD));
                theta_PD = - atan(abs(pos2_PD)/abs(pos1_PD));
            end
        else
            % Second or third quadrant
            if pos2_PD >=0
                % Second quadrant
                theta_PD = pi - atan(abs(pos2_PD)/abs(pos1_PD));
            else
                % Third quadrant
                theta_PD = pi + atan(abs(pos2_PD)/abs(pos1_PD));
            end
        end

        % New target velocity
        vs1_PD = snom*cos(theta_PD);
        vs2_PD = snom*sin(theta_PD);

        % VIRTUAL NOMINAL CONTROLLER (tau1, tau2)
        tau1_nom_PD = - kyd*(vy1 - vs1_PD);
        tau2_nom_PD = - kyd*(vy2 - vs2_PD);

        if (CBF_active == 1)
            % SAFETY FILTERS
            h = (y1 - wp1)^2 + (y2 - wp2)^2 - PTS_Critical^2;
            hdot = 2*(y1 - wp1)*vy1 + 2*(y2 - wp2)*vy2; 
            CONTROL.PARAM.CLASSK = mu2_PTS*CBF_const;
    
            % QUAD PROG COMPONENTS
            A1_qp = 2*(y1 - wp1);
            A2_qp = 2*(y2 - wp2);
    
            if PTS_Active == 1
                % PTS CBF
                psi = hdot + CBF_const*mu2_PTS*h;
                b1_qp = 2*(vy1^2 + vy2^2) + CBF_const*(2*mu2_PTS*mu_PTS/t_nu_active*h + mu2_PTS*hdot) + CBF_const2*mu2_PTS*psi;
                %CONTROL.PARAM.CLASSK = mu2_PTS*CBF_const;
            else
                % HO-CBF
                psi = hdot + CBF_const2*h;
                b1_qp = 2*(vy1^2 + vy2^2) + CBF_const2*hdot + CBF_const2*psi;
                %CONTROL.PARAM.CLASSK = CBF_const;
            end
    
            A_qp = -[A1_qp, A2_qp];
            b_qp = [b1_qp];
            H_qp = [1, 0; 0, 1];
            f_qp = -2*[tau1_nom_PD; tau2_nom_PD];
            x0_qp = [tau1_nom_PD; tau2_nom_PD];
            option_qp = optimoptions('quadprog','Algorithm','active-set','Display','None');            
            [tau_applied, fval_qp, exitval_qp] = quadprog(H_qp, double(f_qp), A_qp, b_qp,[],[],[],[],x0_qp,option_qp);
            tau1_applied = tau_applied(1);
            tau2_applied = tau_applied(2);
            
        else
            tau1_applied = tau1_nom_PD;
            tau2_applied = tau2_nom_PD; 
        end

    else
        % VIRTUAL NOMINAL CONTROLLER (tau1, tau2)
        tau1_applied = - kyd*(vy1 - 0);
        tau2_applied = - kyd*(vy2 - 0);
        tau1_nom_PD = tau1_applied;
        tau2_nom_PD = tau2_applied;
    end

    if abs(tau1_applied) >= tau_max
        tau1_applied = sign(tau1_applied)*tau_max;
    else
        tau1_applied = tau1_applied;
    end

    if abs(tau2_applied) >= tau_max
        tau2_applied = sign(tau2_applied)*tau_max;
    else
        tau2_applied = tau2_applied;
    end
else
     % END OF MISSION
    tau1_nom_PD = - kyd*(vy1 - 0);
    tau2_nom_PD = - kyd*(vy2 - 0);
    tau1_applied = tau1_nom_PD;
    tau2_applied = tau2_nom_PD;
    if abs(tau1_applied) >= tau_max
        tau1_applied = sign(tau1_applied)*tau_max;
    else
        tau1_applied = tau1_applied;
    end

    if abs(tau2_applied) >= tau_max
        tau2_applied = sign(tau2_applied)*tau_max;
    else
        tau2_applied = tau2_applied;
    end
    altitude = 2*10e2;
    rho = altitude + 20.902e6;
    
end

% ESPHERICAL COORDINATES
if y1 >=0
    % First or fourth quadrant
    if y2 >=0
        %First quadrant
        theta_long = atan(abs(y2)/abs(y1));
    else
        % Fourth quadrant
%         theta_long = 2*pi - atan(abs(y2)/abs(y1));
        theta_long = - atan(abs(y2)/abs(y1));
    end
else
    % Second or third quadrant
    if y2 >=0
        % Second quadrant
        theta_long = pi - atan(abs(y2)/abs(y1));
    else
        % Third quadrant
        theta_long = pi + atan(abs(y2)/abs(y1));
    end
end
phi_lat = acos(y1/(rho*cos(theta_long)));

%--------------------------------------------------------------------------
% HEADING CONTROL
%--------------------------------------------------------------------------
% CHANGE OF FRAME FROM XYZ TO NED
sinPOS_Lat = sin(phi_lat);
cosPOS_Lat = cos(phi_lat);
sinPOS_Long = sin(theta_long);
cosPOS_Long = cos(theta_long);

Iner_to_NED = zeros(3,3);
Iner_to_NED(1,1) = - sinPOS_Lat*cosPOS_Long;
Iner_to_NED(2,1) = - sinPOS_Long;
Iner_to_NED(3,1) = - cosPOS_Lat*cosPOS_Long;
Iner_to_NED(1,2) = - sinPOS_Lat*sinPOS_Long;
Iner_to_NED(2,2) = cosPOS_Long;
Iner_to_NED(3,2) = - cosPOS_Lat*sinPOS_Long;
Iner_to_NED(1,3) = cosPOS_Lat;
Iner_to_NED(2,3) = 0;
Iner_to_NED(3,3) = - sinPOS_Lat;

NED_vy = Iner_to_NED*[vy1;vy2;0];
NED_vy1 = NED_vy(1); % NORTH
NED_vy2 = NED_vy(2); % EAST
heading_NED = atan2(NED_vy2,NED_vy1);
heading = atan2(vy2,vy1);

% if NED_vy1 >=0
%     % First or fourth quadrant
%     if NED_vy2 >=0
%         % First quadrant - old 
%         % heading_NED = atan(abs(NED_vy2)/abs(NED_vy1));
%         
%         % With respect to north
%         heading_NED = atan(NED_vy1/NED_vy2) ;
%     else
%         % Fourth quadrant - old
%         % heading_NED = 2*pi - atan(abs(NED_vy2)/abs(NED_vy1));
% 
%         % With respect to north
%         heading_NED = pi/2 + atan(abs(NED_vy1)/abs(NED_vy2));
%     end
% else
%     % Second or third quadrant
%     if NED_vy2 >=0
%         % Second quadrant
%         % heading_NED = pi - atan(abs(NED_vy2)/abs(NED_vy1));
%         % heading_NED = pi - atan(abs(NED_vy1)/abs(NED_vy2));
% 
%         % With respect to north
%         heading_NED = 2*pi - atan(abs(NED_vy1)/abs(NED_vy2));
%     else
%         % Third quadrant
%         % heading_NED = pi + atan(abs(NED_vy2)/abs(NED_vy1));
% %         heading_NED = pi + atan(abs(NED_vy1)/abs(NED_vy2));
% 
%         % With respect to north
%         heading_NED = pi + atan(abs(NED_vy1)/abs(NED_vy2));
%     end
% end
% 
% if vy1 >=0
%     % First or fourth quadrant
%     if vy2 >=0
%         % First quadrant
%         heading = atan(abs(vy2)/abs(vy1));
% 
%         % With respect to north
%         % heading = atan(abs(vy1)/abs(vy2)) + pi;
%     else
%         % Fourth quadrant
%         heading = 2*pi - atan(abs(vy2)/abs(vy1));
%         % heading = - atan(abs(vy1)/abs(vy2));
% 
%         % With respect to north
%         % heading = pi/2 + atan(abs(vy1)/abs(vy2)) + pi;
%     end
% else
%     % Second or third quadrant
%     if vy2 >=0
%         % Second quadrant
%         heading = pi - atan(abs(vy2)/abs(vy1));
% 
%         % With respect to north
%         % heading = 2*pi - atan(abs(vy1)/abs(vy2)) + pi;
%     else
%         % Third quadrant
%         heading = pi + atan(abs(vy2)/abs(vy1));
% 
%         % With respect to north
%         % heading = pi + atan(abs(vy1)/abs(vy2)) + pi;
%     end
% end
%%%%%%%%%%%%%%%%%%%%%%%%%%%%%%%%%%%%%%%%%%%%%%%%%%%%%%%%%%%%%%%%%%%%%%%%%%%
% OUTPUT BUS
%%%%%%%%%%%%%%%%%%%%%%%%%%%%%%%%%%%%%%%%%%%%%%%%%%%%%%%%%%%%%%%%%%%%%%%%%%%
CONTROL.TARGET.WP_INDEX = wp_index;
CONTROL.TARGET.SIMU_END = simu_end;
CONTROL.OUTPUT.TAU1 = tau1_applied;
CONTROL.OUTPUT.TAU2 = tau2_applied;
CONTROL.OUTPUT.LATITUDE = phi_lat;
CONTROL.OUTPUT.LONGITUDE = theta_long;
CONTROL.OUTPUT.HEADING = heading; 
CONTROL.OUTPUT.HEADING_NED = heading_NED; 
CONTROL.PARAM.FLIGHT_STATUS = flight_status;
CONTROL.PARAM.ALTITUDE = altitude;
CONTROL.PARAM.RHO = rho;
CONTROL.PARAM.TIMER = timer;

CONTROL.PARAM.WP_THRESHOLD = wp_Threshold_Flag;
CONTROL.PARAM.WP_TIMER = time_wp_PTS;
CONTROL.PARAM.WP_TIMER_MEM = time_wp_PTS_mem;
CONTROL.PARAM.PTS_ACTIVE_FLAG = PTS_Active;
CONTROL.PARAM.CBF_ACTIVE_FLAG = CBF_active;

CONTROL.PARAM.FVAL = fval_qp;
CONTROL.PARAM.EXITVAL = exitval_qp;

CONTROL.PARAM.CBF_H = h;
CONTROL.PARAM.CBF_PSI = psi;
CONTROL.OUTPUT.TAU1_NOM = tau1_nom_PD;
CONTROL.OUTPUT.TAU2_NOM = tau2_nom_PD;


CONTROL.OUTPUT.NED_VY1 = NED_vy1;
CONTROL.OUTPUT.NED_VY2 = NED_vy2;
return
